simulink model "SelfBalance"  (R2019a)
settings: Solver=VariableStepAuto  StartTime=0.0  StopTime=10  RelTol=1e-3
values from neighbouring files (symbols this model uses):
  A = [0 1;g/l 0]    [PIDtest.m]    (also in SelfBalanceScript.m = [0,1;g/l,0])
  B = [0;1]    [PIDtest.m]    (also in SelfBalanceScript.m)
  C = [1 0]    [PIDtest.m]    (also in PendulumTF.m = pid(Kp,Ki,Kd); SelfBalanceScript.m = [1,0])
  K = [k1;k2]    [PIDtest.m]    (also in SelfBalanceScript.m = lqr(A,B,Q,R))
  x0 = [115;0]    [SelfBalanceScript.m]
settings Model: Creator=jornellq  LastModifiedBy=jornellq

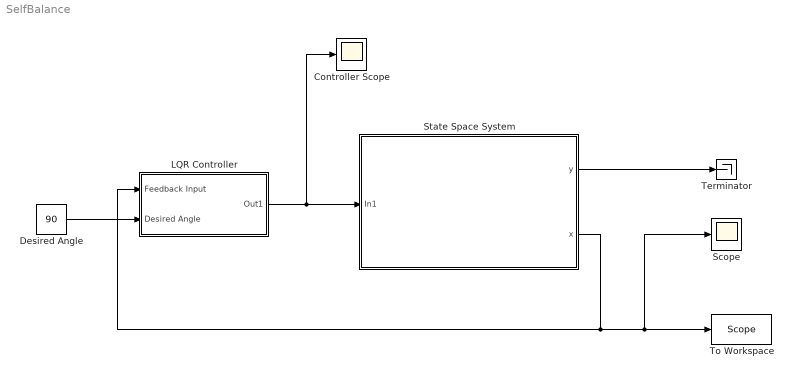
== system SelfBalance ==
  Controller Scope : Scope
  "Desired Angle " : Constant  Value=90
  LQR Controller : Subsystem
  Scope : Scope
  State Space System : Subsystem
  Terminator : Terminator
  To Workspace : ToWorkspace  VariableName=Scope  SampleTime=-1
      settings: Save2DSignal=2-D array (concatenate along first dimension)
  wires:
  State Space System/1("y ") -> Terminator/1
  State Space System/2(x) -> LQR Controller/1(Feedback Input), Scope/1, To Workspace/1
  LQR Controller/1(Out1) -> Controller Scope/1, State Space System/1(In1)
  "Desired Angle "/1 -> LQR Controller/2(Desired Angle)

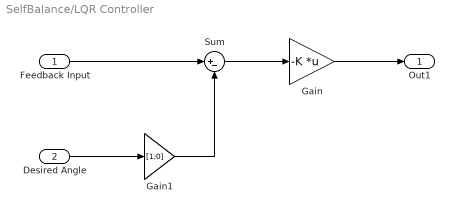
== system SelfBalance/LQR Controller ==
  Feedback Input : Inport
  Desired Angle : Inport  Port=2
  Gain : Gain  Gain=-K  Multiplication=Matrix(K*u)
  Gain1 : Gain  Gain=[1;0]
  Sum : Sum  Inputs=|+-
  Out1 : Outport
  wires:
  Gain/1 -> Out1/1
  Feedback Input/1 -> Sum/1
  Sum/1 -> Gain/1
  Desired Angle/1 -> Gain1/1
  Gain1/1 -> Sum/2

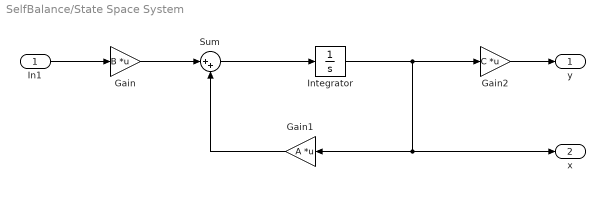
== system SelfBalance/State Space System ==
  In1 : Inport
  Gain : Gain  Gain=B  Multiplication=Matrix(K*u)
  Gain1 : Gain  Gain=A  Multiplication=Matrix(K*u)
  Gain2 : Gain  Gain=C  Multiplication=Matrix(K*u)
  Integrator : Integrator  InitialCondition=x0
  Sum : Sum  Inputs=|++
  "y " : Outport
  x : Outport  Port=2
  wires:
  Gain2/1 -> "y "/1
  In1/1 -> Gain/1
  Gain1/1 -> Sum/2
  Gain/1 -> Sum/1
  Sum/1 -> Integrator/1
  Integrator/1 -> Gain1/1, x/1, Gain2/1
